simulink model "ri_to_c_blk"  (R2019a)
settings: Solver=VariableStepAuto  StartTime=0.0  StopTime=10.0  RelTol=1e-3
libraries: xbsIndex_r4 x1
settings Model: Creator=mybur  LastModifiedBy=mybur

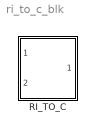
== system ri_to_c_blk ==
  RI_TO_C : Subsystem  mask(ri_to_c){is_async=off}
      mask prompts: is_async "Asynchronous"
      mask help:
      | Concatenates real and imaginary inputs into a complex output.
      | Useful for simplifying interconnects.
      | See also: Complex to Real-Imag (c_to_ri).

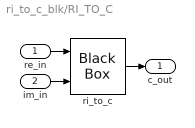
== system ri_to_c_blk/RI_TO_C ==
  re_in : Inport
  im_in : Inport  Port=2
  ri_to_c : xbsIndex_r4/Black Box  init_code=ri_to_c_config  sim_method=ISE Simulator  verbose=off  block_type=blackbox2
  c_out : Outport
  wires:
  ri_to_c/1 -> c_out/1
  re_in/1 -> ri_to_c/1
  im_in/1 -> ri_to_c/2
